simulink model "syringe_motor"  (R2019a)
settings: Solver=VariableStepAuto  StartTime=0.0  StopTime=300  RelTol=1e-3
values from neighbouring files (symbols this model uses):
  filt_const = 5*Ts    (= 0.1)    [syringeparam.m]
  GR = 1/3591.84    (= 0.00027840883781)    [syringeparam.m]
  Ki = 0.0922    [syringeparam.m]
  Kp = 0.0153    [syringeparam.m]
  pin6 = 1    [syringeparam.m]
  pin7 = 0    [syringeparam.m]
  rpm = flow*1083    [syringeparam.m]
  runtime = 55/mm_s    [syringeparam.m]
  Ts = 0.02    [syringeparam.m]
libraries: arduino_io_lib x7
settings Model: Creator=kordelltan  LastModifiedBy=kordelltan

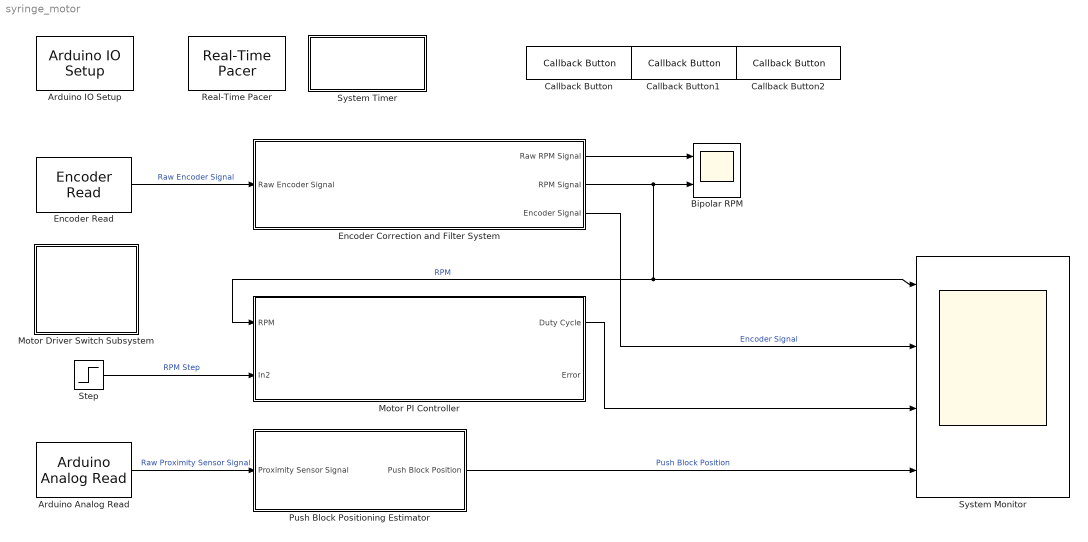
== system syringe_motor ==
  Arduino Analog Read : arduino_io_lib/Arduino Analog Read  arduinoVar=Temporary arduino variable: Arduino1  arduinoPin=5  T=Ts
  Arduino IO Setup : arduino_io_lib/Arduino IO Setup  Priority=3  arduinoVar=Temporary arduino variable: Arduino1  workspaceVarName=a  comPort=/dev/cu.usbmodem14301
  Bipolar RPM : Scope  NumInputPorts=2
  Callback Button : CallbackButton  ButtonText=Infuse
      settings: ClickFcn=|
      | % Set Direction: Forward
      | if pin6 == 1
      |     pin6 = 0;
      | end
      | if pin7 == 0
      |     pin7 = 1;
      | end
      | 
      | % User Input
      | flow = input('ENTER INFUSION RATE (ml/s): ');
      | 
      | % Convert to RPM
      | rpm = flow*1083;
      | mm_s = rpm/130*.6;  % mm per second
      | runtime = 55/mm_s;  % relative runtime needed to infuse maximum
  Callback Button1 : CallbackButton  ButtonText=Reset
      settings: ClickFcn=|
      | % Set Direction: Backwards
      | if pin6 == 0
      |     pin6 = 1;
      | end
      | if pin7 == 1
      |     pin7 = 0;
      | end
      | display('PUMP READY FOR RESET');
  Callback Button2 : CallbackButton  ButtonText=Initialize
      settings: ClickFcn=|
      | % Initialize Motor Driver Pins
      | rpm = 0;
      | pin6 = 1;
      | pin7 = 1;
      | 
      | % Initializing Sampling Time and Signal Filters
      | Ts = 0.02;              % model sample time in seconds
      | GR = 1/3591.84;         % gear ratio 75:1
      | 
      | filt_const = 5*Ts;      % time constant of the first-order filter
      | 
      | % Motor PI Controller Values
      | Kp = 0.0153;
      | Ki = 0.0922;
  Encoder Correction and Filter System : Subsystem
  Encoder Read : arduino_io_lib/Encoder Read  arduinoVar=Temporary arduino variable: Arduino1  encNum=1  pinA=2  pinB=3  DbDl=0  T=0.05
  Motor Driver Switch Subsystem : Subsystem
  Motor PI Controller : Subsystem
  Push Block Positioning Estimator : Subsystem
  Real-Time Pacer : arduino_io_lib/Real-Time Pacer  simTimePerRealTime=1
  Step : Step  Time=0  After=rpm  SampleTime=Ts
  System Monitor : Scope  NumInputPorts=4
  System Timer : Subsystem
  wires:
  Encoder Correction and Filter System/2(RPM Signal) -> Bipolar RPM/2, Motor PI Controller/1(RPM), System Monitor/1  "RPM"
  Encoder Read/1 -> Encoder Correction and Filter System/1(Raw Encoder Signal)  "Raw Encoder Signal"
  Encoder Correction and Filter System/1(Raw RPM Signal) -> Bipolar RPM/1
  Encoder Correction and Filter System/3(Encoder Signal) -> System Monitor/2  "Encoder Signal"
  Step/1 -> Motor PI Controller/2(In2)  "RPM Step"
  Motor PI Controller/1(Duty Cycle) -> System Monitor/3
  Arduino Analog Read/1 -> Push Block Positioning Estimator/1(Proximity Sensor Signal)  "Raw Proximity Sensor Signal"
  Push Block Positioning Estimator/1(Push Block Position) -> System Monitor/4  "Push Block Position"

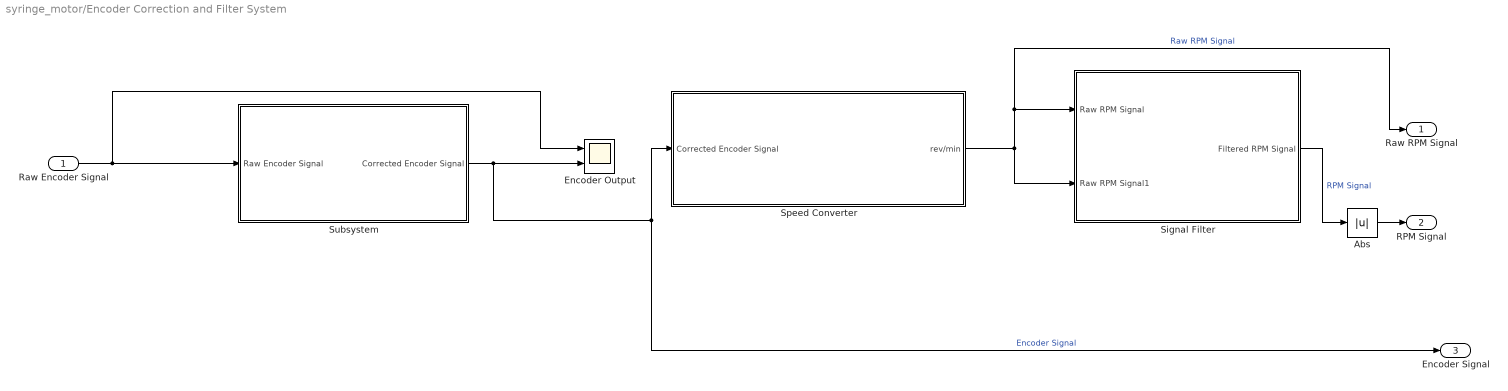
== system syringe_motor/Encoder Correction and Filter System ==
  Raw Encoder Signal : Inport
  Abs : Abs
  Encoder Output : Scope  NumInputPorts=2
  Signal Filter : Subsystem
  "Speed Converter " : Subsystem
  Subsystem : Subsystem
  Raw RPM Signal : Outport
  RPM Signal : Outport  Port=2
  Encoder Signal : Outport  Port=3
  wires:
  Raw Encoder Signal/1 -> Subsystem/1(Raw Encoder Signal), Encoder Output/1
  Signal Filter/1(Filtered RPM Signal) -> Abs/1  "RPM Signal"
  Subsystem/1(Corrected Encoder Signal) -> Encoder Output/2, Encoder Signal/1, "Speed Converter "/1(Corrected Encoder Signal)  "Encoder Signal"
  "Speed Converter "/1(rev/min) -> Signal Filter/2(Raw RPM Signal1), Raw RPM Signal/1, Signal Filter/1(Raw RPM Signal)  "Raw RPM Signal"
  Abs/1 -> RPM Signal/1

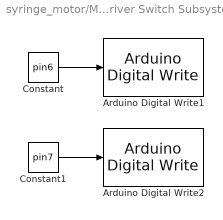
== system syringe_motor/Motor Driver Switch Subsystem ==
  Arduino Digital Write1 : arduino_io_lib/Arduino Digital Write  arduinoVar=Temporary arduino variable: Arduino1  arduinoPin=6  T=0.2
  Arduino Digital Write2 : arduino_io_lib/Arduino Digital Write  arduinoVar=Temporary arduino variable: Arduino1  arduinoPin=7  T=0.2
  Constant : Constant  Value=pin6
  Constant1 : Constant  Value=pin7
  wires:
  Constant1/1 -> Arduino Digital Write2/1
  Constant/1 -> Arduino Digital Write1/1

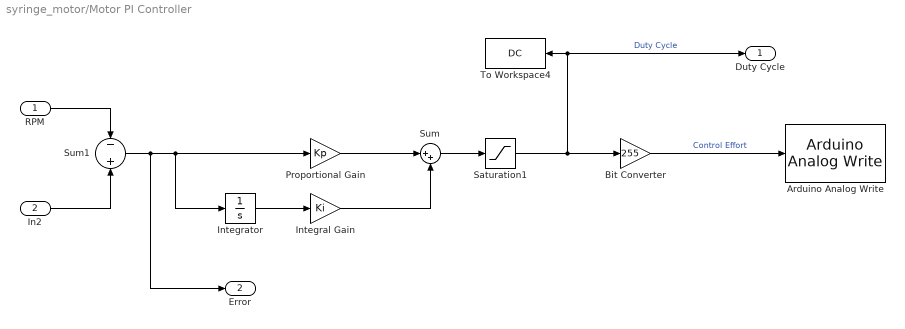
== system syringe_motor/Motor PI Controller ==
  RPM : Inport
  In2 : Inport  Port=2
  Arduino Analog Write : arduino_io_lib/Arduino Analog Write  arduinoVar=Temporary arduino variable: Arduino1  arduinoPin=10  T=Ts
  Bit Converter : Gain  Gain=255
  Integral Gain : Gain  Gain=Ki
  Integrator : Integrator
  Proportional Gain : Gain  Gain=Kp
  Saturation1 : Saturate  UpperLimit=1  LowerLimit=0  SampleTime=Ts
  Sum : Sum  Inputs=|++
  Sum1 : Sum  Inputs=-|+
  To Workspace4 : ToWorkspace  VariableName=DC  SaveFormat=Timeseries  SampleTime=-1
  Duty Cycle : Outport
  Error : Outport  Port=2
  wires:
  Proportional Gain/1 -> Sum/1
  RPM/1 -> Sum1/1
  Bit Converter/1 -> Arduino Analog Write/1  "Control Effort"
  In2/1 -> Sum1/2
  Integrator/1 -> Integral Gain/1
  Saturation1/1 -> Duty Cycle/1, To Workspace4/1, Bit Converter/1  "Duty Cycle"
  Sum1/1 -> Error/1, Integrator/1, Proportional Gain/1
  Integral Gain/1 -> Sum/2
  Sum/1 -> Saturation1/1

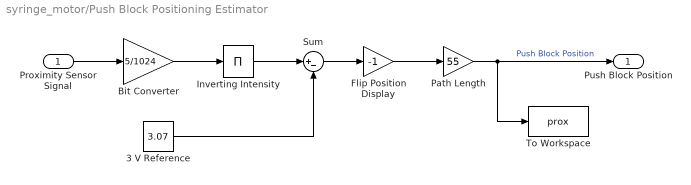
== system syringe_motor/Push Block Positioning Estimator ==
  Proximity Sensor Signal : Inport
  3 V Reference : Constant  Value=3.07
  Bit Converter : Gain  Gain=5/1024
  Flip Position Display : Gain  Gain=-1
  Inverting Intensity : Product  Inputs=1
  Path Length : Gain  Gain=55
  Sum : Sum  Inputs=|+-
  To Workspace : ToWorkspace  VariableName=prox  SaveFormat=Timeseries  SampleTime=-1
  Push Block Position : Outport
  wires:
  Flip Position Display/1 -> Path Length/1
  Path Length/1 -> Push Block Position/1, To Workspace/1  "Push Block Position"
  3 V Reference/1 -> Sum/2
  Inverting Intensity/1 -> Sum/1
  Proximity Sensor Signal/1 -> Bit Converter/1
  Bit Converter/1 -> Inverting Intensity/1
  Sum/1 -> Flip Position Display/1

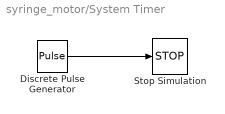
== system syringe_motor/System Timer ==
  Discrete Pulse Generator : DiscretePulseGenerator  Period=fix(runtime/Ts)  PulseWidth=fix(runtime/Ts)  PhaseDelay=fix(runtime/Ts)  SampleTime=Ts
  Stop Simulation : Stop
  wires:
  Discrete Pulse Generator/1 -> Stop Simulation/1

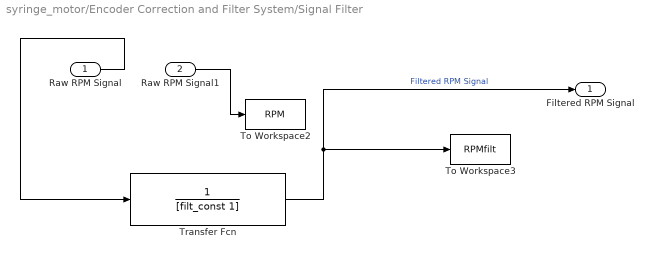
== system syringe_motor/Encoder Correction and Filter System/Signal Filter ==
  Raw RPM Signal : Inport
  Raw RPM Signal1 : Inport  Port=2
  To Workspace2 : ToWorkspace  VariableName=RPM  SaveFormat=Timeseries  SampleTime=-1
  To Workspace3 : ToWorkspace  VariableName=RPMfilt  SaveFormat=Timeseries  SampleTime=-1
  Transfer Fcn : TransferFcn  Denominator=[filt_const 1]
  Filtered RPM Signal : Outport
  wires:
  Raw RPM Signal1/1 -> To Workspace2/1
  Raw RPM Signal/1 -> Transfer Fcn/1
  Transfer Fcn/1 -> Filtered RPM Signal/1, To Workspace3/1  "Filtered RPM Signal"

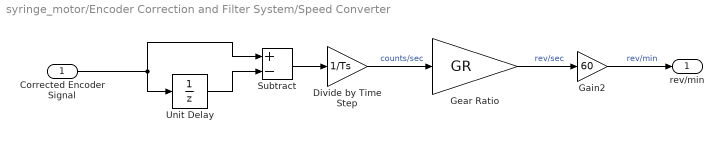
== system syringe_motor/Encoder Correction and Filter System/Speed Converter  ==
  Corrected Encoder Signal : Inport
  Divide by Time Step : Gain  Gain=1/Ts
  Gain2 : Gain  Gain=60
  Gear Ratio : Gain  Gain=GR
  Subtract : Sum  Inputs=+-
  Unit Delay : UnitDelay  SampleTime=-1  HasFrameUpgradeWarning=on
  rev/min : Outport
  wires:
  Unit Delay/1 -> Subtract/2
  Gain2/1 -> rev/min/1  "rev/min"
  Divide by Time Step/1 -> Gear Ratio/1  "counts/sec"
  Subtract/1 -> Divide by Time Step/1
  Gear Ratio/1 -> Gain2/1  "rev/sec"
  Corrected Encoder Signal/1 -> Subtract/1, Unit Delay/1

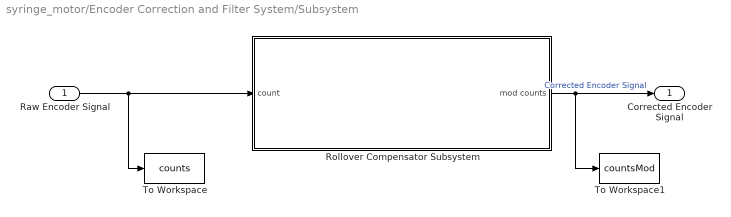
== system syringe_motor/Encoder Correction and Filter System/Subsystem ==
  Raw Encoder Signal : Inport
  Rollover Compensator Subsystem : Subsystem
  To Workspace : ToWorkspace  VariableName=counts  SaveFormat=Timeseries  SampleTime=-1
  To Workspace1 : ToWorkspace  VariableName=countsMod  SaveFormat=Timeseries  SampleTime=-1
  Corrected Encoder Signal : Outport
  wires:
  Raw Encoder Signal/1 -> Rollover Compensator Subsystem/1(count), To Workspace/1
  Rollover Compensator Subsystem/1("mod counts ") -> Corrected Encoder Signal/1, To Workspace1/1  "Corrected Encoder Signal"

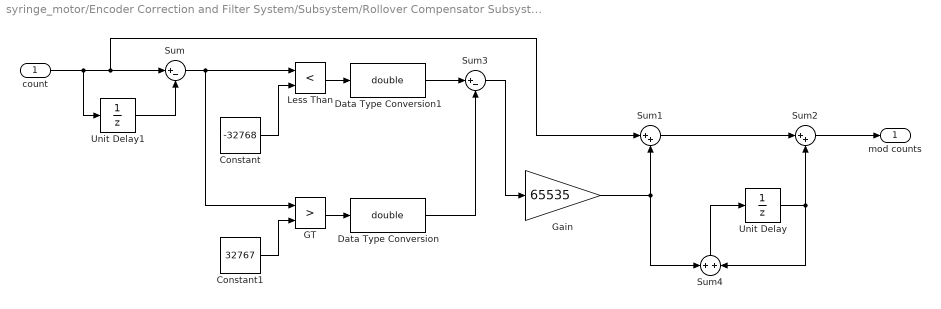
== system syringe_motor/Encoder Correction and Filter System/Subsystem/Rollover Compensator Subsystem ==
  count : Inport
  Constant : Constant  Value=-32768
  Constant1 : Constant  Value=32767
  Data Type Conversion : DataTypeConversion  OutDataTypeStr=double
  Data Type Conversion1 : DataTypeConversion  OutDataTypeStr=double
  GT : RelationalOperator  Operator=>  OutDataTypeStr=boolean  RndMeth=Simplest
  Gain : Gain  Gain=65535
  Less Than : RelationalOperator  Operator=<  OutDataTypeStr=boolean  RndMeth=Simplest
  Sum : Sum  Inputs=|+-
  Sum1 : Sum  Inputs=|++
  Sum2 : Sum  Inputs=|++
  Sum3 : Sum  Inputs=|+-
  Sum4 : Sum  Inputs=+|+
  Unit Delay : UnitDelay  SampleTime=-1  HasFrameUpgradeWarning=on
  Unit Delay1 : UnitDelay  SampleTime=-1  HasFrameUpgradeWarning=on
  "mod counts " : Outport
  wires:
  GT/1 -> Data Type Conversion/1
  Constant1/1 -> GT/2
  Sum4/1 -> Unit Delay/1
  Gain/1 -> Sum1/2, Sum4/1
  Data Type Conversion1/1 -> Sum3/1
  Sum2/1 -> "mod counts "/1
  count/1 -> Unit Delay1/1, Sum1/1, Sum/1
  Constant/1 -> Less Than/2
  Unit Delay1/1 -> Sum/2
  Sum/1 -> GT/1, Less Than/1
  Data Type Conversion/1 -> Sum3/2
  Less Than/1 -> Data Type Conversion1/1
  Unit Delay/1 -> Sum4/2, Sum2/2
  Sum1/1 -> Sum2/1
  Sum3/1 -> Gain/1
